simulink model "ADCS_testing"  (R2021a)
settings: Solver=FixedStepAuto  StartTime=0.0  StopTime=200  RelTol=1e-3  EnableMultiTasking=on
libraries: arduinolib x7, simulink_extras x2, arduinosensorlib x1
settings Model: SILPILModeSetting=veronly  ExtModeTrigDuration=2  Creator=admin  LastModifiedBy=admin
settings OptimizationCC: EnhancedBackFolding=on  PassReuseOutputArgsAs=Individual arguments  ZeroExternalMemoryAtStartup=off  ZeroInternalMemoryAtStartup=off  MaxStackSize=64  OptimizeBlockOrder=speed  DifferentSizesBufferReuse=on  OptimizationCustomize=off  EfficientTunableParamExpr=on
settings DebuggingCC: ParameterTunabilityLossMsg=error
settings HardwareCC: ProdBitPerPointer=32  ProdBitPerSizeT=32  ProdBitPerPtrDiffT=32  ProdLargestAtomicInteger=Long  ProdLargestAtomicFloat=Double  ProdWordSize=32  ProdHWDeviceType=ARM Compatible->ARM Cortex
settings SFSimCC: MATLABDynamicMemAlloc=off
settings RTWCC: SystemTargetFile=ert.tlc  HardwareBoard=Arduino Due  TLCOptions="-aInlineSetEventsForThisBaseRateFcn=TLC_FALSE -aSuppressMultiTaskScheduler=TLC_FALSE   -aRateBasedStepFcn=1"  TemplateMakefile=ert_default_tmf  Toolchain=Arduino ARM  BuildConfiguration=Faster Runs
settings CodeAppCC: ForceParamTrailComments=on  IgnoreCustomStorageClasses=off  OperatorAnnotations=on  SimulinkDataObjDesc=on  SFDataObjDesc=on  InsertBlockDesc=on
settings ERTTargetCC: SupportContinuousTime=on  SupportVariableSizeSignals=on  ExtModeTransport=3  ExtModeStaticAlloc=on  ExtModeStaticAllocSize=24576  ExtModeMexFile=ext_xcp  ExtModeIntrfLevel=Level2 - Open

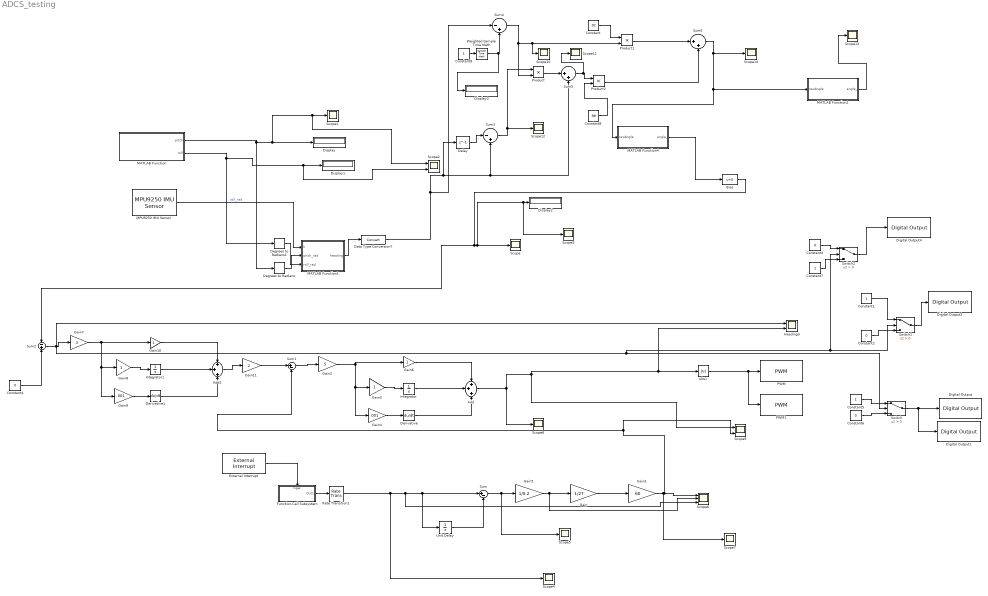
== system ADCS_testing ==
  Abs1 : Abs
  Add : Sum  Inputs=+++
  Add1 : Sum  Inputs=+++
  Bias : Bias
  Constant : Constant  Value=.02
  Constant{1,5,7,9} (4 alike) : Constant
  Constant{2..4,6} (4 alike) : Constant  Value=0
  Constant8 : Constant  Value=.98
  Data Type Conversion7 : DataTypeConversion
  Degrees to Radians : simulink_extras/Transformations/Degrees to Radians
  Degrees to Radians1 : simulink_extras/Transformations/Degrees to Radians
  Delay : Delay  DelayLength=1
  Derivative : Derivative  CoefficientInTFapproximation=.2
  Derivative1 : Derivative
  Digital Output : arduinolib/Digital Output  pinNumber=6  Direction=output  blockPlatform=arduino
  Digital Output1 : arduinolib/Digital Output  pinNumber=7  Direction=output  blockPlatform=arduino
  Digital Output2 : arduinolib/Digital Output  pinNumber=8  Direction=output  blockPlatform=arduino
  Digital Output4 : arduinolib/Digital Output  pinNumber=9  Direction=output  blockPlatform=arduino
  Display{,1..3} (4 alike) : Display
  External Interrupt : arduinolib/External Interrupt  Pin=2  PullUp=off  Mode=RISING  InterruptSimulationInput=off
      settings: SourceProductBaseCode=ARDUINO
  Function-Call Subsystem : Subsystem  TreatAsAtomicUnit=on
  Gain : Gain  Gain=1/27
  Gain1 : Gain  Gain=60
  Gain{3,6,8,10} (4 alike) : Gain
  Gain11 : Gain  Gain=.2
  Gain2 : Gain  Gain=.5
  Gain4 : Gain  Gain=.001
  Gain5 : Gain  Gain=1/0.2
  Gain7 : Gain  Gain=.3
  Gain9 : Gain  Gain=.001
  Heading3 : Scope  NumInputPorts=2
  Integrator : Integrator
  Integrator1 : Integrator
  MATLAB Function : MATLAB Function  TreatAsAtomicUnit=on  SystemSampleTime=1/100
  MATLAB Function1 : MATLAB Function  TreatAsAtomicUnit=on
  MATLAB Function2 : MATLAB Function  TreatAsAtomicUnit=on
  MATLAB Function4 : MATLAB Function  TreatAsAtomicUnit=on
  MPU9250 IMU Sensor : arduinosensorlib/MPU9250 IMU Sensor  SlaveAddress=0x68  Accel=off  AngularRate=off  Ak8963Field=on  Temperature=off  Status=off  EulerAngles=off  Quat=off  AccelRange=2G  Acceldlpf=218.1 Hz  GyroRange=250 dps  Gyrodlpf=250 Hz  DmpOdr=200 Hz  SampleTime=-1
      settings: SourceProductBaseCode=ARDUINO
  PWM : arduinolib/PWM  pinNumber=4  frequencyType=Default  desiredFrequency=490.2  achievableFrequency=490.2
  PWM1 : arduinolib/PWM  pinNumber=5  frequencyType=Default  desiredFrequency=490.2  achievableFrequency=490.2
  Product : Product
  Product1 : Product
  Product2 : Product
  Rate Transition1 : RateTransition  Deterministic=off
  Scope{,1,3..5,7..8,10..14} (12 alike) : Scope
  Scope2 : Scope  NumInputPorts=2
  Scope6 : Scope  NumInputPorts=3
  Scope9 : Scope  NumInputPorts=2
  Sum : Sum  Inputs=|+-
  Sum1 : Sum  Inputs=|+-
  Sum2 : Sum  Inputs=-+
  Sum3 : Sum  Inputs=|-+
  Sum4 : Sum  Inputs=|-+
  Sum5 : Sum  Inputs=|++
  Sum6 : Sum  Inputs=|++
  Switch : Switch  Criteria=u2 > Threshold
  Switch1 : Switch  Criteria=u2 > Threshold
  Switch2 : Switch  Criteria=u2 > Threshold
  Unit Delay : UnitDelay  SampleTime=-1  HasFrameUpgradeWarning=on
  Weighted Sample Time Math : SampleTimeMath  TsampMathOp=*
  wires:
  Constant8/1 -> Product2/2
  Sum5/1 -> Scope11/1, Product2/1
  Constant9/1 -> Weighted Sample Time Math/1
  Constant/1 -> Product1/1
  Sum6/1 -> MATLAB Function4/1(rawAngle), MATLAB Function2/1(rawAngle), Scope14/1
  Product2/1 -> Sum6/2
  Sum3/1 -> Product/1, Scope12/1
  Product1/1 -> Sum6/1
  Constant2/1 -> Switch1/3
  Gain3/1 -> Integrator/1
  MATLAB Function/2(roll) -> Degrees to Radians1/1, Scope2/2, Display1/1
  Constant1/1 -> Switch1/1
  External Interrupt/1 -> Function-Call Subsystem/Trigger
  Sum1/1 -> Gain2/1
  Sum2/1 -> Switch2/2, Switch1/2, Switch/2, Heading3/1, Gain7/1
  Weighted Sample Time Math/1 -> Display3/1, Sum4/2
  Product/1 -> Sum5/1
  Bias/1 -> Scope3/1, Display2/1, Scope/1, Sum2/1
  Function-Call Subsystem/1(Out1) -> Rate Transition1/1
  Rate Transition1/1 -> Scope6/3, Unit Delay/1, Sum/1, Scope4/1
  Gain6/1 -> Add/1
  Gain9/1 -> Derivative1/1
  Gain7/1 -> Gain9/1, Gain8/1, Gain10/1
  Gain10/1 -> Add1/1
  Add1/1 -> Gain11/1
  Derivative1/1 -> Add1/3
  Constant4/1 -> Sum2/2
  Derivative/1 -> Add/3
  Unit Delay/1 -> Sum/2
  Gain1/1 -> Scope7/1, Scope6/1, Scope9/2, Sum1/2
  Integrator/1 -> Add/2
  MATLAB Function1/1(heading) -> Data Type Conversion7/1
  MATLAB Function/1(pitch) -> Degrees to Radians/1, Scope2/1, Scope1/1, Display/1
  Constant6/1 -> Switch/3
  Constant5/1 -> Switch/1
  MPU9250 IMU Sensor/1 -> MATLAB Function1/1(h)  "roll_rad"
  Integrator1/1 -> Add1/2
  Switch/1 -> Digital Output1/1, Digital Output/1
  Sum4/1 -> Scope10/1, Product1/2, Product/2
  Abs1/1 -> PWM1/1, PWM/1
  Gain11/1 -> Sum1/1
  Gain2/1 -> Gain4/1, Gain3/1, Gain6/1
  Switch2/1 -> Digital Output4/1
  Gain8/1 -> Integrator1/1
  Constant7/1 -> Switch2/3
  Degrees to Radians/1 -> MATLAB Function1/2(pitch_rad)
  Degrees to Radians1/1 -> MATLAB Function1/3(roll_rad)
  Switch1/1 -> Digital Output2/1
  Gain/1 -> Gain1/1
  Gain4/1 -> Derivative/1
  Delay/1 -> Sum3/1
  Data Type Conversion7/1 -> Sum4/1, Delay/1, Sum5/2, Sum3/2
  MATLAB Function4/1(angle_) -> Bias/1
  Gain5/1 -> Scope6/2, Gain/1
  Add/1 -> Abs1/1, Heading3/2, Scope9/1, Scope8/1
  Sum/1 -> Scope5/1, Gain5/1
  Constant3/1 -> Switch2/1
  MATLAB Function2/1(angle_) -> Scope13/1

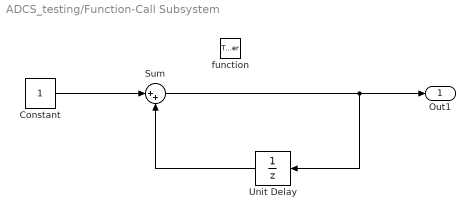
== system ADCS_testing/Function-Call Subsystem ==
  function : TriggerPort  TriggerType=function-call  VariantControl=(inherit)
  Constant : Constant  SampleTime=-1
  Sum : Sum  Inputs=|++
  Unit Delay : UnitDelay  SampleTime=-1  HasFrameUpgradeWarning=on
  Out1 : Outport  VectorParamsAs1DForOutWhenUnconnected=off
  wires:
  Unit Delay/1 -> Sum/2
  Constant/1 -> Sum/1
  Sum/1 -> Unit Delay/1, Out1/1

== matlab function ADCS_testing/MATLAB Function2 ==
  data: rawAngle input; angle_ output
function angle_ = constrainerHeading(rawAngle)
angle_ = rawAngle;
    if rawAngle > 360 
        angle_ = rawAngle - 360;
    elseif angle_ < 0
       angle_ =  rawAngle + 360;
    end
end

== matlab function ADCS_testing/MATLAB Function ==
  data: pitch output; roll output
function [pitch, roll] = calculatePitchRoll()

% This function reads acceleration and angular velocity from an IMU sensor
% and calculates its orientation by finding out pitch and roll. In this
% application MPU9250 sensor is used. However, it could be replaced with
% any other IMU sensor as well.

persistent arduinoObj imuObj
persistent prevTimestamp
persistent pitchAngle rollAngle
persistent pitchAccelOffset rollAccelOffset pitchGyroOffset rollGyroOffset

% Output
roll = 0;
pitch = 0;

if isempty(arduinoObj)
    arduinoObj = arduino();
end
if isempty(imuObj)
    imuObj = mpu9250(arduinoObj);
end

% x -> longitudinal axis or N axis or roll axis
% y -> transverse axis or E axis or pitch axis
% z -> vertical axis or  D axis or yaw axis
if isempty(pitchAccelOffset)
pitchAccelOffset = 0;
pitchGyroOffset = 0;
rollAccelOffset = 0;
rollGyroOffset = 0;
prevTimestamp = 0;

% Calculate the average offset error produced by accelerometer and gyroscope.
count = 100;
for i = 1:count
    if i == count
        [accel, gyro, ~, timestamp] = read(imuObj);
        prevTimestamp = timestamp;
    else
        [accel, gyro] = read(imuObj);
    end
    pitchAccelOffset = pitchAccelOffset + atan2(accel(1), sqrt(accel(2)*accel(2) + accel(3)*accel(3)));
    rollAccelOffset = rollAccelOffset + atan2(-accel(2), sqrt(accel(1)*accel(1) + accel(3)*accel(3)));
    pitchGyroOffset = pitchGyroOffset + gyro(2);
    rollGyroOffset = rollGyroOffset + gyro(1);
end

pitchAccelOffset = pitchAccelOffset/count;
rollAccelOffset = rollAccelOffset/count;
pitchGyroOffset = pitchGyroOffset/count;
rollGyroOffset = rollGyroOffset/count;
end

if isempty(pitchAngle)
    pitchAngle = 0;
end

if isempty(rollAngle)
    rollAngle = 0;
end

% Using complementary filter to fuse accelerometer and gyroscope data.
% Filter coefficient should be tuned to improve result
filterCoeff = 0.98;

[accel, gyro, ~, timestamp] = read(imuObj);
% Calculate pitch and roll from acceleration values and remove offset
accelPitchAngle = atan2(accel(1), sqrt(accel(2)*accel(2) + accel(3)*accel(3))) - pitchAccelOffset;
accelRollAngle = atan2(-accel(2), sqrt(accel(1)*accel(1) + accel(3)*accel(3))) - rollAccelOffset;
% Subtract the offset values calculated at the beginning
gyro(1) = gyro(1) - rollGyroOffset;
gyro(2) = gyro(2) - pitchGyroOffset;
gyroPitchAngleDiff = gyro(2)*(timestamp - prevTimestamp);
gyroRollAngleDiff = gyro(1)*(timestamp - prevTimestamp);
prevTimestamp = timestamp;

% Use complementary filter to fuse accelerometer and gyroscope data
pitchAngle = filterCoeff*(pitchAngle + gyroPitchAngleDiff) + (1 - filterCoeff)*accelPitchAngle;
rollAngle = filterCoeff*(rollAngle + gyroRollAngleDiff) + (1 - filterCoeff)*accelRollAngle;

% sensor object returns angular velocity in radians/s. Converting pitch and
% roll angles into degree
pitch = pitchAngle*180/pi;
roll = rollAngle*180/pi;

== matlab function ADCS_testing/MATLAB Function1 ==
  data: heading output; h input; pitch_rad input; roll_rad input
function heading = mag2Heading(h,pitch_rad,roll_rad)

 h = normalize(h,'norm');
 mag_x = h(1)*cos(pitch_rad) + h(2)*sin(roll_rad)*sin(pitch_rad) + h(3)*cos(roll_rad)*sin(pitch_rad);
 mag_y = h(2) * cos(roll_rad) - h(3) * sin(roll_rad);
 yawAngle = 180 * atan2(-mag_y,mag_x)/pi;
 
 heading = yawAngle;

== matlab function ADCS_testing/MATLAB Function4 ==
  data: rawAngle input; angle_ output
function angle_ = constrainerHeading(rawAngle)
angle_ = rawAngle;
    if rawAngle > 360 
        angle_ = rawAngle - 360;
    elseif angle_ < 0
       angle_ =  rawAngle + 360;
    end
end
